simulink model "Parallel_n64"  (R2012b)
settings: Solver=VariableStepDiscrete  StartTime=0.0  StopTime=TotalIterations  RelTol=1e-3
values from neighbouring files (symbols this model uses):
  bp = 12    [ConfigValidate.m]
  bpSNMemory = bp    (= 12)    [ConfigValidate.m]
  IterationsOrdering = 4000    [ConfigValidate.m]
  MaxCoordDistance = (abs(max(wx) - min(wx))+abs(max(wy) - min(wy)))^2    [ConfigValidate.m]
  N_limit = 0.01    [ConfigValidate.m]
  nBits = 9    [ConfigValidate.m]
  nBitsNSmemories = (ceil(log2(TotalIterations)))    [ConfigValidate.m]
  S_limit = 1    [ConfigValidate.m]
  SourceNodes = 2000    [ConfigValidate.m]
  ts = 1    [ConfigValidate.m]
  w1 = rand(1,Neurons)    [ConfigValidate.m]
  w2 = rand(1,Neurons)    [ConfigValidate.m]
  wx = zeros(1,Neurons)    [ConfigValidate.m]
  wy = zeros(1,Neurons)    [ConfigValidate.m]
  x1 = rand(SourceNodes,1)    [ConfigValidate.m]
  x2 = rand(SourceNodes,1)    [ConfigValidate.m]
libraries: xbsIndex_r4 x6367, dspsrcs4 x2, dspstat3 x2
(part 1 of 28)
settings Model: Creator=Leonardo  LastModifiedBy=leona

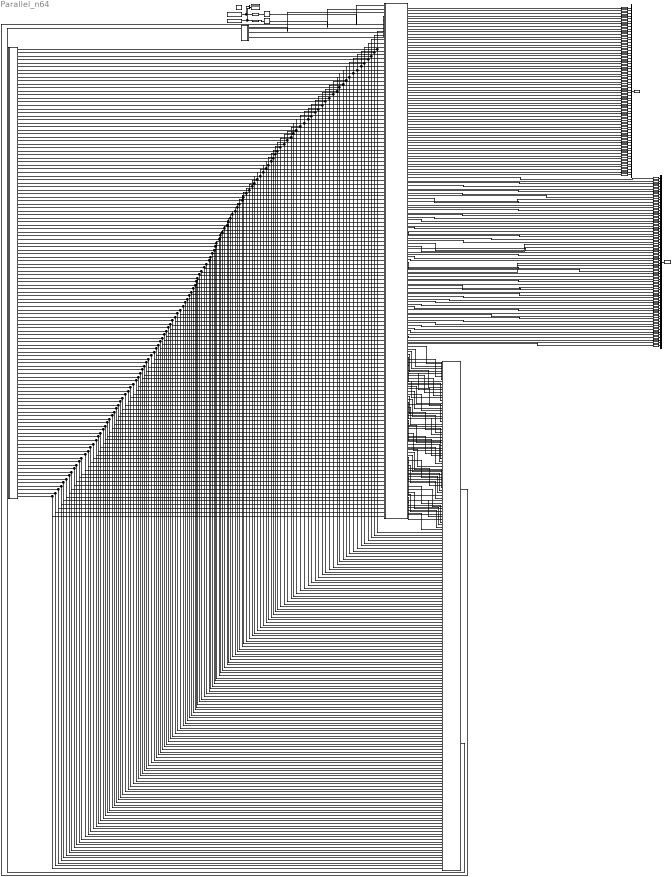
== system Parallel_n64 ==
  " System Generator" : xbsIndex_r4/ System Generator  Tag=genX  xilinxfamily=virtex6  part=xc6vlx240t  speed=-1  package=ff1156  synthesis_tool=XST  clock_wrapper=Clock Enables  directory=./n64d2nt  proj_type=Project Navigator  Synth_file=XST Defaults  Impl_file=ISE Defaults  testbench=off  simulink_period=ts  sysclk_period=10  dcm_input_clock_period=10  incr_netlist=off  trim_vbits=Everywhere in SubSystem  dbl_ovrd=According to Block Masks  core_generation=According to Block Masks  run_coregen=off  deprecated_control=off  eval_field=0  block_type=sysgen
  Coordinates : Subsystem
  Display2 : Display
  Gateway Out{1,3..75,77..128} (126 alike) : xbsIndex_r4/Gateway Out  inherit_from_input=off  hdl_port=off  timing_constraint=None  locs_specified=off  LOCs={}  UseAsDAC=off  DACChannel='1'  block_type=gatewayout
  Gateway Out2 : xbsIndex_r4/Gateway Out  inherit_from_input=off  hdl_port=on  timing_constraint=None  locs_specified=off  LOCs={}  UseAsDAC=off  DACChannel='1'  block_type=gatewayout
  Gateway Out76 : xbsIndex_r4/Gateway Out  inherit_from_input=off  hdl_port=on  timing_constraint=None  locs_specified=off  LOCs={}  UseAsDAC=off  DACChannel='1'  block_type=gatewayout
  Mux1 : Mux  Inputs=64
  Mux3 : Mux  Inputs=2
  Mux5 : Mux  Inputs=64
  Neurons : Subsystem
  Signal From Workspace : dspsrcs4/Signal From Workspace  X=x1(1:SourceNodes)  Ts=ts  nsamps=1  OutputAfterFinalValue=Cyclic repetition  ignoreOrWarnInputAndFrameLengths=off
  Signal From Workspace1 : dspsrcs4/Signal From Workspace  X=x2(1:SourceNodes)  Ts=ts  nsamps=1  OutputAfterFinalValue=Cyclic repetition  ignoreOrWarnInputAndFrameLengths=off
  TimeSeries_Functions : Subsystem
  To Workspace : ToWorkspace  VariableName=w1_histH  SampleTime=ts
  To Workspace1 : ToWorkspace  VariableName=w2_histH  SampleTime=ts
  WiningNeuronFinder1 : Subsystem
  delay_vX11 : xbsIndex_r4/Register  init=x1(1)  rst=off  en=off  dbl_ovrd=off  block_type=register
  delay_vX12 : xbsIndex_r4/Register  init=x2(1)  rst=off  en=off  dbl_ovrd=off  block_type=register
  "vX11_in " : xbsIndex_r4/Gateway In  gui_display_data_type=Fixed-point  arith_type="Signed  (2's comp)"  n_bits=nb  bin_pt=bp  preci_type=Single  exp_width=8  frac_width=24  quantization="Round  (unbiased: +/- Inf)"  overflow=Saturate  period=ts  dbl_ovrd=off  timing_constraint=None  locs_specified=off  LOCs={}  UseAsADC=off  ADCChannel='1'  inherit_from_input=off  hdl_port=on  block_type=gatewayin
  vX12_in : xbsIndex_r4/Gateway In  gui_display_data_type=Fixed-point  arith_type="Signed  (2's comp)"  n_bits=nb  bin_pt=bp  preci_type=Single  exp_width=8  frac_width=24  quantization="Round  (unbiased: +/- Inf)"  overflow=Saturate  period=ts  dbl_ovrd=off  timing_constraint=None  locs_specified=off  LOCs={}  UseAsADC=off  ADCChannel='1'  inherit_from_input=off  hdl_port=on  block_type=gatewayin
  wires:
  Signal From Workspace/1 -> Mux3/1, "vX11_in "/1
  Signal From Workspace1/1 -> Mux3/2, vX12_in/1
  Mux3/1 -> Display2/1
  vX12_in/1 -> delay_vX12/1
  delay_vX12/1 -> Neurons/2(vX12)
  TimeSeries_Functions/1(S) -> Neurons/3(S)
  TimeSeries_Functions/2(N) -> Neurons/4(N)
  TimeSeries_Functions/3(MemControl) -> Neurons/5(memControl)
  Mux5/1 -> To Workspace/1
  "vX11_in "/1 -> delay_vX11/1
  delay_vX11/1 -> Neurons/1(vX11)
  Neurons/61(w1n61) -> Gateway Out64/1
  Neurons/34(w1n34) -> Gateway Out27/1
  Neurons/35(w1n35) -> Gateway Out26/1
  Neurons/31(w1n31) -> Gateway Out35/1
  Neurons/33(w1n33) -> Gateway Out36/1
  Neurons/32(w1n32) -> Gateway Out34/1
  Neurons/40(w1n40) -> Gateway Out44/1
  Neurons/45(w1n45) -> Gateway Out48/1
  Neurons/36(w1n36) -> Gateway Out28/1
  Neurons/44(w1n44) -> Gateway Out46/1
  Neurons/39(w1n39) -> Gateway Out42/1
  Neurons/43(w1n43) -> Gateway Out47/1
  Neurons/42(w1n42) -> Gateway Out45/1
  Neurons/37(w1n37) -> Gateway Out41/1
  Neurons/38(w1n38) -> Gateway Out37/1
  Neurons/41(w1n41) -> Gateway Out43/1
  Neurons/27(w1n27) -> Gateway Out30/1
  Neurons/26(w1n26) -> Gateway Out25/1
  Neurons/29(w1n29) -> Gateway Out31/1
  Neurons/28(w1n28) -> Gateway Out32/1
  Neurons/30(w1n30) -> Gateway Out33/1
  Neurons/64(w1n64) -> Gateway Out63/1
  Neurons/63(w1n63) -> Gateway Out61/1
  Neurons/62(w1n62) -> Gateway Out62/1
  Neurons/6(w1n6) -> Gateway Out6/1
  Neurons/9(w1n9) -> Gateway Out9/1
  Neurons/10(w1n10) -> Gateway Out11/1
  Neurons/1(w1n1) -> Gateway Out2/1
  Neurons/2(w1n2) -> Gateway Out1/1
  Neurons/3(w1n3) -> Gateway Out3/1
  Neurons/4(w1n4) -> Gateway Out5/1
  Neurons/5(w1n5) -> Gateway Out4/1
  Neurons/7(w1n7) -> Gateway Out8/1
  Neurons/8(w1n8) -> Gateway Out7/1
  Neurons/23(w1n23) -> Gateway Out14/1
  Neurons/12(w1n12) -> Gateway Out12/1
  Neurons/11(w1n11) -> Gateway Out10/1
  Neurons/14(w1n14) -> Gateway Out13/1
  Neurons/19(w1n19) -> Gateway Out23/1
  Neurons/24(w1n24) -> Gateway Out16/1
  Neurons/13(w1n13) -> Gateway Out17/1
  Neurons/15(w1n15) -> Gateway Out18/1
  Neurons/18(w1n18) -> Gateway Out21/1
  Neurons/17(w1n17) -> Gateway Out19/1
  Neurons/20(w1n20) -> Gateway Out22/1
  Neurons/22(w1n22) -> Gateway Out15/1
  Neurons/25(w1n25) -> Gateway Out29/1
  Neurons/16(w1n16) -> Gateway Out20/1
  Neurons/21(w1n21) -> Gateway Out24/1
  Neurons/54(w1n54) -> Gateway Out51/1
  Neurons/51(w1n51) -> Gateway Out54/1
  Neurons/52(w1n52) -> Gateway Out50/1
  Neurons/48(w1n48) -> Gateway Out40/1
  Neurons/50(w1n50) -> Gateway Out52/1
  Neurons/46(w1n46) -> Gateway Out39/1
  Neurons/49(w1n49) -> Gateway Out53/1
  Neurons/47(w1n47) -> Gateway Out38/1
  Neurons/53(w1n53) -> Gateway Out49/1
  Neurons/57(w1n57) -> Gateway Out60/1
  Neurons/58(w1n58) -> Gateway Out56/1
  Neurons/60(w1n60) -> Gateway Out57/1
  Neurons/59(w1n59) -> Gateway Out55/1
  Neurons/56(w1n56) -> Gateway Out58/1
  Neurons/55(w1n55) -> Gateway Out59/1
  Mux1/1 -> To Workspace1/1
  Neurons/85(w2n21) -> Gateway Out81/1
  Neurons/87(w2n23) -> Gateway Out70/1
  Neurons/86(w2n22) -> Gateway Out71/1
  Neurons/89(w2n25) -> Gateway Out86/1
  Neurons/88(w2n24) -> Gateway Out72/1
  Neurons/75(w2n11) -> Gateway Out66/1
  Neurons/78(w2n14) -> Gateway Out69/1
  Neurons/77(w2n13) -> Gateway Out73/1
  Neurons/79(w2n15) -> Gateway Out74/1
  Neurons/76(w2n12) -> Gateway Out68/1
  Neurons/69(w2n5) -> Gateway Out98/1
  Neurons/100(w2n36) -> Gateway Out85/1
  Neurons/103(w2n39) -> Gateway Out101/1
  Neurons/104(w2n40) -> Gateway Out103/1
  Neurons/101(w2n37) -> Gateway Out100/1
  Neurons/102(w2n38) -> Gateway Out95/1
  Neurons/109(w2n45) -> Gateway Out107/1
  Neurons/108(w2n44) -> Gateway Out105/1
  Neurons/107(w2n43) -> Gateway Out106/1
  Neurons/105(w2n41) -> Gateway Out102/1
  Neurons/106(w2n42) -> Gateway Out104/1
  Neurons/80(w2n16) -> Gateway Out77/1
  Neurons/83(w2n19) -> Gateway Out80/1
  Neurons/82(w2n18) -> Gateway Out78/1
  Neurons/81(w2n17) -> Gateway Out75/1
  Neurons/84(w2n20) -> Gateway Out79/1
  Neurons/70(w2n6) -> Gateway Out120/1
  Neurons/71(w2n7) -> Gateway Out127/1
  Neurons/74(w2n10) -> Gateway Out67/1
  Neurons/72(w2n8) -> Gateway Out126/1
  Neurons/73(w2n9) -> Gateway Out128/1
  Neurons/90(w2n26) -> Gateway Out82/1
  Neurons/93(w2n29) -> Gateway Out89/1
  Neurons/94(w2n30) -> Gateway Out91/1
  Neurons/91(w2n27) -> Gateway Out88/1
  Neurons/92(w2n28) -> Gateway Out90/1
  Neurons/67(w2n3) -> Gateway Out87/1
  Neurons/110(w2n46) -> Gateway Out97/1
  Neurons/112(w2n48) -> Gateway Out99/1
  Neurons/111(w2n47) -> Gateway Out96/1
  Neurons/113(w2n49) -> Gateway Out113/1
  Neurons/116(w2n52) -> Gateway Out110/1
  Neurons/115(w2n51) -> Gateway Out114/1
  Neurons/118(w2n54) -> Gateway Out111/1
  Neurons/114(w2n50) -> Gateway Out112/1
  Neurons/119(w2n55) -> Gateway Out119/1
  Neurons/117(w2n53) -> Gateway Out108/1
  Neurons/66(w2n2) -> Gateway Out65/1
  Neurons/65(w2n1) -> Gateway Out76/1
  Neurons/95(w2n31) -> Gateway Out93/1
  Neurons/96(w2n32) -> Gateway Out92/1
  Neurons/97(w2n33) -> Gateway Out94/1
  Neurons/99(w2n35) -> Gateway Out83/1
  Neurons/98(w2n34) -> Gateway Out84/1
  Neurons/120(w2n56) -> Gateway Out118/1
  Neurons/124(w2n60) -> Gateway Out117/1
  Neurons/121(w2n57) -> Gateway Out121/1
  Neurons/122(w2n58) -> Gateway Out116/1
  Neurons/123(w2n59) -> Gateway Out115/1
  Neurons/128(w2n64) -> Gateway Out124/1
  Neurons/125(w2n61) -> Gateway Out125/1
  Neurons/126(w2n62) -> Gateway Out123/1
  Neurons/127(w2n63) -> Gateway Out122/1
  Neurons/68(w2n4) -> Gateway Out109/1
  Gateway Out2/1 -> Mux5/1
  Gateway Out1/1 -> Mux5/2
  Gateway Out3/1 -> Mux5/3
  Gateway Out5/1 -> Mux5/4
  Gateway Out6/1 -> Mux5/6
  Gateway Out4/1 -> Mux5/5
  Gateway Out8/1 -> Mux5/7
  Gateway Out10/1 -> Mux5/11
  Gateway Out9/1 -> Mux5/9
  Gateway Out7/1 -> Mux5/8
  Gateway Out11/1 -> Mux5/10
  Gateway Out12/1 -> Mux5/12
  Gateway Out13/1 -> Mux5/14
  Gateway Out22/1 -> Mux5/20
  Gateway Out17/1 -> Mux5/13
  Gateway Out20/1 -> Mux5/16
  Gateway Out14/1 -> Mux5/23
  Gateway Out15/1 -> Mux5/22
  Gateway Out16/1 -> Mux5/24
  Gateway Out19/1 -> Mux5/17
  Gateway Out18/1 -> Mux5/15
  Gateway Out21/1 -> Mux5/18
  Gateway Out23/1 -> Mux5/19
  Gateway Out24/1 -> Mux5/21
  Gateway Out25/1 -> Mux5/26
  Gateway Out27/1 -> Mux5/34
  Gateway Out26/1 -> Mux5/35
  Gateway Out28/1 -> Mux5/36
  Gateway Out36/1 -> Mux5/33
  Gateway Out30/1 -> Mux5/27
  Gateway Out32/1 -> Mux5/28
  Gateway Out29/1 -> Mux5/25
  Gateway Out35/1 -> Mux5/31
  Gateway Out31/1 -> Mux5/29
  Gateway Out34/1 -> Mux5/32
  Gateway Out33/1 -> Mux5/30
  Gateway Out45/1 -> Mux5/42
  Gateway Out43/1 -> Mux5/41
  Gateway Out44/1 -> Mux5/40
  Gateway Out46/1 -> Mux5/44
  Gateway Out39/1 -> Mux5/46
  Gateway Out41/1 -> Mux5/37
  Gateway Out40/1 -> Mux5/48
  Gateway Out38/1 -> Mux5/47
  Gateway Out42/1 -> Mux5/39
  Gateway Out37/1 -> Mux5/38
  Gateway Out48/1 -> Mux5/45
  Gateway Out47/1 -> Mux5/43
  Gateway Out51/1 -> Mux5/54
  Gateway Out52/1 -> Mux5/50
  Gateway Out54/1 -> Mux5/51
  Gateway Out49/1 -> Mux5/53
  Gateway Out50/1 -> Mux5/52
  Gateway Out53/1 -> Mux5/49
  Gateway Out60/1 -> Mux5/57
  Gateway Out57/1 -> Mux5/60
  Gateway Out56/1 -> Mux5/58
  Gateway Out59/1 -> Mux5/55
  Gateway Out55/1 -> Mux5/59
  Gateway Out58/1 -> Mux5/56
  Gateway Out61/1 -> Mux5/63
  Gateway Out64/1 -> Mux5/61
  Gateway Out63/1 -> Mux5/64
  Gateway Out62/1 -> Mux5/62
  Gateway Out66/1 -> Mux1/11
  Gateway Out69/1 -> Mux1/14
  Gateway Out67/1 -> Mux1/10
  Gateway Out70/1 -> Mux1/23
  Gateway Out68/1 -> Mux1/12
  Gateway Out73/1 -> Mux1/13
  Gateway Out72/1 -> Mux1/24
  Gateway Out75/1 -> Mux1/17
  Gateway Out71/1 -> Mux1/22
  Gateway Out74/1 -> Mux1/15
  Gateway Out79/1 -> Mux1/20
  Gateway Out80/1 -> Mux1/19
  Gateway Out76/1 -> Mux1/1
  Gateway Out77/1 -> Mux1/16
  Gateway Out78/1 -> Mux1/18
  Gateway Out84/1 -> Mux1/34
  Gateway Out85/1 -> Mux1/36
  Gateway Out82/1 -> Mux1/26
  Gateway Out81/1 -> Mux1/21
  Gateway Out83/1 -> Mux1/35
  Gateway Out88/1 -> Mux1/27
  Gateway Out90/1 -> Mux1/28
  Gateway Out89/1 -> Mux1/29
  Gateway Out86/1 -> Mux1/25
  Gateway Out87/1 -> Mux1/3
  Gateway Out92/1 -> Mux1/32
  Gateway Out93/1 -> Mux1/31
  Gateway Out94/1 -> Mux1/33
  Gateway Out91/1 -> Mux1/30
  Gateway Out95/1 -> Mux1/38
  Gateway Out96/1 -> Mux1/47
  Gateway Out98/1 -> Mux1/5
  Gateway Out97/1 -> Mux1/46
  Gateway Out99/1 -> Mux1/48
  Gateway Out101/1 -> Mux1/39
  Gateway Out100/1 -> Mux1/37
  Gateway Out65/1 -> Mux1/2
  Gateway Out102/1 -> Mux1/41
  Gateway Out113/1 -> Mux1/49
  Gateway Out106/1 -> Mux1/43
  Gateway Out111/1 -> Mux1/54
  Gateway Out114/1 -> Mux1/51
  Gateway Out115/1 -> Mux1/59
  Gateway Out105/1 -> Mux1/44
  Gateway Out110/1 -> Mux1/52
  Gateway Out104/1 -> Mux1/42
  Gateway Out109/1 -> Mux1/4
  Gateway Out107/1 -> Mux1/45
  Gateway Out112/1 -> Mux1/50
  Gateway Out103/1 -> Mux1/40
  Gateway Out108/1 -> Mux1/53
  Gateway Out127/1 -> Mux1/7
  Gateway Out128/1 -> Mux1/9
  Gateway Out124/1 -> Mux1/64
  Gateway Out120/1 -> Mux1/6
  Gateway Out121/1 -> Mux1/57
  Gateway Out122/1 -> Mux1/63
  Gateway Out116/1 -> Mux1/58
  Gateway Out118/1 -> Mux1/56
  Gateway Out125/1 -> Mux1/61
  Gateway Out123/1 -> Mux1/62
  Gateway Out126/1 -> Mux1/8
  Gateway Out117/1 -> Mux1/60
  Gateway Out119/1 -> Mux1/55
  Neurons/139(dist_n11) -> WiningNeuronFinder1/11(dist_k11)
  Neurons/143(dist_n15) -> WiningNeuronFinder1/15(dist_k15)
  Neurons/142(dist_n14) -> WiningNeuronFinder1/14(dist_k14)
  Neurons/140(dist_n12) -> WiningNeuronFinder1/12(dist_k12)
  Neurons/141(dist_n13) -> WiningNeuronFinder1/13(dist_k13)
  Neurons/150(dist_n22) -> WiningNeuronFinder1/22(dist_k22)
  Neurons/153(dist_n25) -> WiningNeuronFinder1/25(dist_k25)
  Neurons/152(dist_n24) -> WiningNeuronFinder1/24(dist_k24)
  Neurons/151(dist_n23) -> WiningNeuronFinder1/23(dist_k23)
  Neurons/149(dist_n21) -> WiningNeuronFinder1/21(dist_k21)
  Neurons/144(dist_n16) -> WiningNeuronFinder1/16(dist_k16)
  Neurons/145(dist_n17) -> WiningNeuronFinder1/17(dist_k17)
  Neurons/148(dist_n20) -> WiningNeuronFinder1/20(dist_k20)
  Neurons/147(dist_n19) -> WiningNeuronFinder1/19(dist_k19)
  Neurons/146(dist_n18) -> WiningNeuronFinder1/18(dist_k18)
  Neurons/129(dist_n1) -> WiningNeuronFinder1/1(dist_k1)
  Neurons/169(dist_n41) -> WiningNeuronFinder1/41(dist_k41)
  Neurons/172(dist_n44) -> WiningNeuronFinder1/44(dist_k44)
  Neurons/171(dist_n43) -> WiningNeuronFinder1/43(dist_k43)
  Neurons/173(dist_n45) -> WiningNeuronFinder1/45(dist_k45)
  Neurons/170(dist_n42) -> WiningNeuronFinder1/42(dist_k42)
  Neurons/175(dist_n47) -> WiningNeuronFinder1/47(dist_k47)
  Neurons/174(dist_n46) -> WiningNeuronFinder1/46(dist_k46)
  Neurons/176(dist_n48) -> WiningNeuronFinder1/48(dist_k48)
  Neurons/178(dist_n50) -> WiningNeuronFinder1/50(dist_k50)
  Neurons/177(dist_n49) -> WiningNeuronFinder1/49(dist_k49)
  Neurons/131(dist_n3) -> WiningNeuronFinder1/3(dist_k3)
  Neurons/132(dist_n4) -> WiningNeuronFinder1/4(dist_k4)
  Neurons/155(dist_n27) -> WiningNeuronFinder1/27(dist_k27)
  Neurons/156(dist_n28) -> WiningNeuronFinder1/28(dist_k28)
  Neurons/157(dist_n29) -> WiningNeuronFinder1/29(dist_k29)
  Neurons/158(dist_n30) -> WiningNeuronFinder1/30(dist_k30)
  Neurons/154(dist_n26) -> WiningNeuronFinder1/26(dist_k26)
  Neurons/179(dist_n51) -> WiningNeuronFinder1/51(dist_k51)
  Neurons/181(dist_n53) -> WiningNeuronFinder1/53(dist_k53)
  Neurons/188(dist_n60) -> WiningNeuronFinder1/60(dist_k60)
  Neurons/182(dist_n54) -> WiningNeuronFinder1/54(dist_k54)
  Neurons/183(dist_n55) -> WiningNeuronFinder1/55(dist_k55)
  Neurons/180(dist_n52) -> WiningNeuronFinder1/52(dist_k52)
  Neurons/186(dist_n58) -> WiningNeuronFinder1/58(dist_k58)
  Neurons/184(dist_n56) -> WiningNeuronFinder1/56(dist_k56)
  Neurons/185(dist_n57) -> WiningNeuronFinder1/57(dist_k57)
  Neurons/187(dist_n59) -> WiningNeuronFinder1/59(dist_k59)
  Neurons/130(dist_n2) -> WiningNeuronFinder1/2(dist_k2)
  Neurons/159(dist_n31) -> WiningNeuronFinder1/31(dist_k31)
  Neurons/163(dist_n35) -> WiningNeuronFinder1/35(dist_k35)
  Neurons/161(dist_n33) -> WiningNeuronFinder1/33(dist_k33)
  Neurons/160(dist_n32) -> WiningNeuronFinder1/32(dist_k32)
  Neurons/162(dist_n34) -> WiningNeuronFinder1/34(dist_k34)
  Neurons/168(dist_n40) -> WiningNeuronFinder1/40(dist_k40)
  Neurons/166(dist_n38) -> WiningNeuronFinder1/38(dist_k38)
  Neurons/165(dist_n37) -> WiningNeuronFinder1/37(dist_k37)
  Neurons/164(dist_n36) -> WiningNeuronFinder1/36(dist_k36)
  Neurons/167(dist_n39) -> WiningNeuronFinder1/39(dist_k39)
  Neurons/189(dist_n61) -> WiningNeuronFinder1/61(dist_k61)
  Neurons/190(dist_n62) -> WiningNeuronFinder1/62(dist_k62)
  Neurons/191(dist_n63) -> WiningNeuronFinder1/63(dist_k63)
  Neurons/192(dist_n64) -> WiningNeuronFinder1/64(dist_k64)
  Neurons/133(dist_n5) -> WiningNeuronFinder1/5(dist_k5)
  Neurons/138(dist_n10) -> WiningNeuronFinder1/10(dist_k10)
  Neurons/137(dist_n9) -> WiningNeuronFinder1/9(dist_k9)
  Neurons/134(dist_n6) -> WiningNeuronFinder1/6(dist_k6)
  Neurons/136(dist_n8) -> WiningNeuronFinder1/8(dist_k8)
  Neurons/135(dist_n7) -> WiningNeuronFinder1/7(dist_k7)
  WiningNeuronFinder1/1(WinningNeuron_wx) -> Neurons/6(wx_win)
  WiningNeuronFinder1/2(WinningNeuron_wy) -> Neurons/7(wy_win)
  Coordinates/128(wy64) -> WiningNeuronFinder1/192(wy_64), Neurons/135(wy64)
  Coordinates/127(wx64) -> WiningNeuronFinder1/191(wx_64), Neurons/134(wx64)
  Coordinates/126(wy63) -> WiningNeuronFinder1/190(wy_63), Neurons/133(wy63)
  Coordinates/125(wx63) -> WiningNeuronFinder1/189(wx_63), Neurons/132(wx63)
  Coordinates/124(wy62) -> WiningNeuronFinder1/188(wy_62), Neurons/131(wy62)
  Coordinates/123(wx62) -> WiningNeuronFinder1/187(wx_62), Neurons/130(wx62)
  Coordinates/122(wy61) -> WiningNeuronFinder1/186(wy_61), Neurons/129(wy61)
  Coordinates/121(wx61) -> WiningNeuronFinder1/185(wx_61), Neurons/128(wx61)
  Coordinates/120(wy60) -> WiningNeuronFinder1/184(wy_60), Neurons/127(wy60)
  Coordinates/119(wx60) -> WiningNeuronFinder1/183(wx_60), Neurons/126(wx60)
  Coordinates/118(wy59) -> WiningNeuronFinder1/182(wy_59), Neurons/125(wy59)
  Coordinates/117(wx59) -> WiningNeuronFinder1/181(wx_59), Neurons/124(wx59)
  Coordinates/116(wy58) -> WiningNeuronFinder1/180(wy_58), Neurons/123(wy58)
  Coordinates/115(wx58) -> WiningNeuronFinder1/179(wx_58), Neurons/122(wx58)
  Coordinates/114(wy57) -> WiningNeuronFinder1/178(wy_57), Neurons/121(wy57)
  Coordinates/113(wx57) -> WiningNeuronFinder1/177(wx_57), Neurons/120(wx57)
  Coordinates/112(wy56) -> WiningNeuronFinder1/176(wy_56), Neurons/119(wy56)
  Coordinates/111(wx56) -> WiningNeuronFinder1/175(wx_56), Neurons/118(wx56)
  Coordinates/110(wy55) -> WiningNeuronFinder1/174(wy_55), Neurons/117(wy55)
  Coordinates/109(wx55) -> WiningNeuronFinder1/173(wx_55), Neurons/116(wx55)
  Coordinates/108(wy54) -> WiningNeuronFinder1/172(wy_54), Neurons/115(wy54)
  Coordinates/107(wx54) -> WiningNeuronFinder1/171(wx_54), Neurons/114(wx54)
  Coordinates/106(wy53) -> WiningNeuronFinder1/170(wy_53), Neurons/113(wy53)
  Coordinates/105(wx53) -> WiningNeuronFinder1/169(wx_53), Neurons/112(wx53)
  Coordinates/104(wy52) -> WiningNeuronFinder1/168(wy_52), Neurons/111(wy52)
  Coordinates/103(wx52) -> WiningNeuronFinder1/167(wx_52), Neurons/110(wx52)
  Coordinates/102(wy51) -> WiningNeuronFinder1/166(wy_51), Neurons/109(wy51)
  Coordinates/101(wx51) -> WiningNeuronFinder1/165(wx_51), Neurons/108(wx51)
  Coordinates/100(wy50) -> WiningNeuronFinder1/164(wy_50), Neurons/107(wy50)
  Coordinates/99(wx50) -> WiningNeuronFinder1/163(wx_50), Neurons/106(wx50)
  Coordinates/98(wy49) -> WiningNeuronFinder1/162(wy_49), Neurons/105(wy49)
  Coordinates/97(wx49) -> WiningNeuronFinder1/161(wx_49), Neurons/104(wx49)
  Coordinates/96(wy48) -> WiningNeuronFinder1/160(wy_48), Neurons/103(wy48)
  Coordinates/95(wx48) -> WiningNeuronFinder1/159(wx_48), Neurons/102(wx48)
  Coordinates/93(wx47) -> WiningNeuronFinder1/157(wx_47), Neurons/100(wx47)
  Coordinates/92(wy46) -> WiningNeuronFinder1/156(wy_46), Neurons/99(wy46)
  Coordinates/91(wx46) -> WiningNeuronFinder1/155(wx_46), Neurons/98(wx46)
  Coordinates/90(wy45) -> WiningNeuronFinder1/154(wy_45), Neurons/97(wy45)
  Coordinates/88(wy44) -> WiningNeuronFinder1/152(wy_44), Neurons/95(wy44)
  Coordinates/87(wx44) -> WiningNeuronFinder1/151(wx_44), Neurons/94(wx44)
  Coordinates/86(wy43) -> WiningNeuronFinder1/150(wy_43), Neurons/93(wy43)
  Coordinates/85(wx43) -> WiningNeuronFinder1/149(wx_43), Neurons/92(wx43)
  Coordinates/84(wy42) -> WiningNeuronFinder1/148(wy_42), Neurons/91(wy42)
  Coordinates/83(wx42) -> WiningNeuronFinder1/147(wx_42), Neurons/90(wx42)
  Coordinates/81(wx41) -> WiningNeuronFinder1/145(wx_41), Neurons/88(wx41)
  Coordinates/80(wy40) -> WiningNeuronFinder1/144(wy_40), Neurons/87(wy40)
  Coordinates/79(wx40) -> WiningNeuronFinder1/143(wx_40), Neurons/86(wx40)
  Coordinates/78(wy39) -> WiningNeuronFinder1/142(wy_39), Neurons/85(wy39)
  Coordinates/77(wx39) -> WiningNeuronFinder1/141(wx_39), Neurons/84(wx39)
  Coordinates/76(wy38) -> WiningNeuronFinder1/140(wy_38), Neurons/83(wy38)
  Coordinates/75(wx38) -> WiningNeuronFinder1/139(wx_38), Neurons/82(wx38)
  Coordinates/74(wy37) -> WiningNeuronFinder1/138(wy_37), Neurons/81(wy37)
  Coordinates/73(wx37) -> WiningNeuronFinder1/137(wx_37), Neurons/80(wx37)
  Coordinates/72(wy36) -> WiningNeuronFinder1/136(wy_36), Neurons/79(wy36)
  Coordinates/71(wx36) -> WiningNeuronFinder1/135(wx_36), Neurons/78(wx36)
  Coordinates/70(wy35) -> WiningNeuronFinder1/134(wy_35), Neurons/77(wy35)
  Coordinates/69(wx35) -> WiningNeuronFinder1/133(wx_35), Neurons/76(wx35)
  Coordinates/68(wy34) -> WiningNeuronFinder1/132(wy_34), Neurons/75(wy34)
  Coordinates/67(wx34) -> WiningNeuronFinder1/131(wx_34), Neurons/74(wx34)
  Coordinates/66(wy33) -> WiningNeuronFinder1/130(wy_33), Neurons/73(wy33)
  Coordinates/65(wx33) -> WiningNeuronFinder1/129(wx_33), Neurons/72(wx33)
  Coordinates/63(wx32) -> WiningNeuronFinder1/127(wx_32), Neurons/70(wx32)
  Coordinates/62(wy31) -> WiningNeuronFinder1/126(wy_31), Neurons/69(wy31)
  Coordinates/61(wx31) -> WiningNeuronFinder1/125(wx_31), Neurons/68(wx31)
  Coordinates/59(wx30) -> WiningNeuronFinder1/123(wx_30), Neurons/66(wx30)
  Coordinates/58(wy29) -> WiningNeuronFinder1/122(wy_29), Neurons/65(wy29)
  Coordinates/57(wx29) -> WiningNeuronFinder1/121(wx_29), Neurons/64(wx29)
  Coordinates/56(wy28) -> WiningNeuronFinder1/120(wy_28), Neurons/63(wy28)
  Coordinates/54(wy27) -> WiningNeuronFinder1/118(wy_27), Neurons/61(wy27)
  Coordinates/53(wx27) -> WiningNeuronFinder1/117(wx_27), Neurons/60(wx27)
  Coordinates/52(wy26) -> WiningNeuronFinder1/116(wy_26), Neurons/59(wy26)
  Coordinates/51(wx26) -> WiningNeuronFinder1/115(wx_26), Neurons/58(wx26)
  Coordinates/50(wy25) -> WiningNeuronFinder1/114(wy_25), Neurons/57(wy25)
  Coordinates/49(wx25) -> WiningNeuronFinder1/113(wx_25), Neurons/56(wx25)
  Coordinates/48(wy24) -> WiningNeuronFinder1/112(wy_24), Neurons/55(wy24)
  Coordinates/47(wx24) -> WiningNeuronFinder1/111(wx_24), Neurons/54(wx24)
  Coordinates/46(wy23) -> WiningNeuronFinder1/110(wy_23), Neurons/53(wy23)
  Coordinates/45(wx23) -> WiningNeuronFinder1/109(wx_23), Neurons/52(wx23)
  Coordinates/43(wx22) -> WiningNeuronFinder1/107(wx_22), Neurons/50(wx22)
  Coordinates/42(wy21) -> WiningNeuronFinder1/106(wy_21), Neurons/49(wy21)
  Coordinates/41(wx21) -> WiningNeuronFinder1/105(wx_21), Neurons/48(wx21)
  Coordinates/40(wy20) -> WiningNeuronFinder1/104(wy_20), Neurons/47(wy20)
  Coordinates/39(wx20) -> WiningNeuronFinder1/103(wx_20), Neurons/46(wx20)
  Coordinates/38(wy19) -> WiningNeuronFinder1/102(wy_19), Neurons/45(wy19)
  Coordinates/37(wx19) -> WiningNeuronFinder1/101(wx_19), Neurons/44(wx19)
  Coordinates/36(wy18) -> WiningNeuronFinder1/100(wy_18), Neurons/43(wy18)
  Coordinates/35(wx18) -> WiningNeuronFinder1/99(wx_18), Neurons/42(wx18)
  Coordinates/34(wy17) -> WiningNeuronFinder1/98(wy_17), Neurons/41(wy17)
  Coordinates/32(wy16) -> WiningNeuronFinder1/96(wy_16), Neurons/39(wy16)
  Coordinates/31(wx16) -> WiningNeuronFinder1/95(wx_16), Neurons/38(wx16)
  Coordinates/30(wy15) -> WiningNeuronFinder1/94(wy_15), Neurons/37(wy15)
  Coordinates/29(wx15) -> WiningNeuronFinder1/93(wx_15), Neurons/36(wx15)
  Coordinates/28(wy14) -> WiningNeuronFinder1/92(wy_14), Neurons/35(wy14)
  Coordinates/27(wx14) -> WiningNeuronFinder1/91(wx_14), Neurons/34(wx14)
  Coordinates/26(wy13) -> WiningNeuronFinder1/90(wy_13), Neurons/33(wy13)
  Coordinates/25(wx13) -> WiningNeuronFinder1/89(wx_13), Neurons/32(wx13)
  Coordinates/23(wx12) -> WiningNeuronFinder1/87(wx_12), Neurons/30(wx12)
  Coordinates/22(wy11) -> WiningNeuronFinder1/86(wy_11), Neurons/29(wy11)
  Coordinates/21(wx11) -> WiningNeuronFinder1/85(wx_11), Neurons/28(wx11)
  Coordinates/20(wy10) -> WiningNeuronFinder1/84(wy_10), Neurons/27(wy10)
  Coordinates/19(wx10) -> WiningNeuronFinder1/83(wx_10), Neurons/26(wx10)
  Coordinates/18(wy9) -> WiningNeuronFinder1/82(wy_9), Neurons/25(wy9)
  Coordinates/17(wx9) -> WiningNeuronFinder1/81(wx_9), Neurons/24(wx9)
  Coordinates/16(wy8) -> WiningNeuronFinder1/80(wy_8), Neurons/23(wy8)
  Coordinates/15(wx8) -> WiningNeuronFinder1/79(wx_8), Neurons/22(wx8)
  Coordinates/14(wy7) -> WiningNeuronFinder1/78(wy_7), Neurons/21(wy7)
  Coordinates/13(wx7) -> WiningNeuronFinder1/77(wx_7), Neurons/20(wx7)
  Coordinates/12(wy6) -> WiningNeuronFinder1/76(wy_6), Neurons/19(wy6)
  Coordinates/11(wx6) -> WiningNeuronFinder1/75(wx_6), Neurons/18(wx6)
  Coordinates/10(wy5) -> WiningNeuronFinder1/74(wy_5), Neurons/17(wy5)
  Coordinates/9(wx5) -> WiningNeuronFinder1/73(wx_5), Neurons/16(wx5)
  Coordinates/8(wy4) -> WiningNeuronFinder1/72(wy_4), Neurons/15(wy4)
  Coordinates/7(wx4) -> WiningNeuronFinder1/71(wx_4), Neurons/14(wx4)
  Coordinates/6(wy3) -> WiningNeuronFinder1/70(wy_3), Neurons/13(wy3)
  Coordinates/4(wy2) -> WiningNeuronFinder1/68(wy_2), Neurons/11(wy2)
  Coordinates/2(wy1) -> WiningNeuronFinder1/66(wy_1), Neurons/9(wy1)
  Coordinates/1(wx1) -> WiningNeuronFinder1/65(wx_1), Neurons/8(wx1)
  Coordinates/3(wx2) -> WiningNeuronFinder1/67(wx_2), Neurons/10(wx2)
  Coordinates/5(wx3) -> WiningNeuronFinder1/69(wx_3), Neurons/12(wx3)
  Coordinates/24(wy12) -> WiningNeuronFinder1/88(wy_12), Neurons/31(wy12)
  Coordinates/33(wx17) -> WiningNeuronFinder1/97(wx_17), Neurons/40(wx17)
  Coordinates/44(wy22) -> WiningNeuronFinder1/108(wy_22), Neurons/51(wy22)
  Coordinates/55(wx28) -> WiningNeuronFinder1/119(wx_28), Neurons/62(wx28)
  Coordinates/60(wy30) -> WiningNeuronFinder1/124(wy_30), Neurons/67(wy30)
  Coordinates/64(wy32) -> WiningNeuronFinder1/128(wy_32), Neurons/71(wy32)
  Coordinates/82(wy41) -> WiningNeuronFinder1/146(wy_41), Neurons/89(wy41)
  Coordinates/89(wx45) -> WiningNeuronFinder1/153(wx_45), Neurons/96(wx45)
  Coordinates/94(wy47) -> WiningNeuronFinder1/158(wy_47), Neurons/101(wy47)
